simulink model "lungmodel"  (R2021a)
settings: Solver=ode8  StartTime=0.0  StopTime=10.0  FixedStep=1e-2  RelTol=1e-3
settings Model: Creator=Asus  LastModifiedBy=Asus

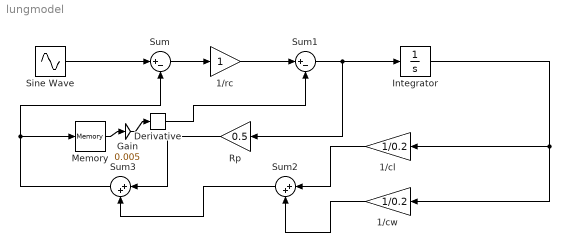
== system lungmodel ==
  1/cl : Gain  Gain=1/0.2
  1/cw : Gain  Gain=1/0.2
  1/rc : Gain
  Derivative : Derivative
  Gain : Gain  Gain=0.005
  Integrator : Integrator
  Memory : Memory
  Rp : Gain  Gain=0.5
  Sine Wave : Sin  SampleTime=0
  Sum : Sum  Inputs=|+-
  Sum1 : Sum  Inputs=|+-
  Sum2 : Sum  Inputs=|++
  Sum3 : Sum  Inputs=|++
  wires:
  Sine Wave/1 -> Sum/1
  Sum/1 -> 1/rc/1
  1/rc/1 -> Sum1/1
  Sum1/1 -> Rp/1, Integrator/1
  Integrator/1 -> 1/cw/1, 1/cl/1
  1/cl/1 -> Sum2/1
  1/cw/1 -> Sum2/2
  Sum2/1 -> Sum3/2
  Rp/1 -> Sum3/1
  Sum3/1 -> Memory/1, Sum/2
  Memory/1 -> Gain/1
  Gain/1 -> Derivative/1
  Derivative/1 -> Sum1/2
